simulink model "launch_control"  (R2023b)
settings: Solver=VariableStepAuto  StartTime=0.0  StopTime=10.0  RelTol=1e-3
settings Model: Creator=no  LastModifiedBy=no

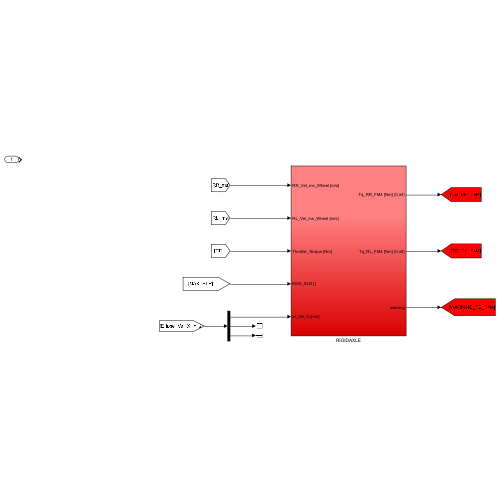
[thumbnail: Simulink's stored preview of the top-level diagram]
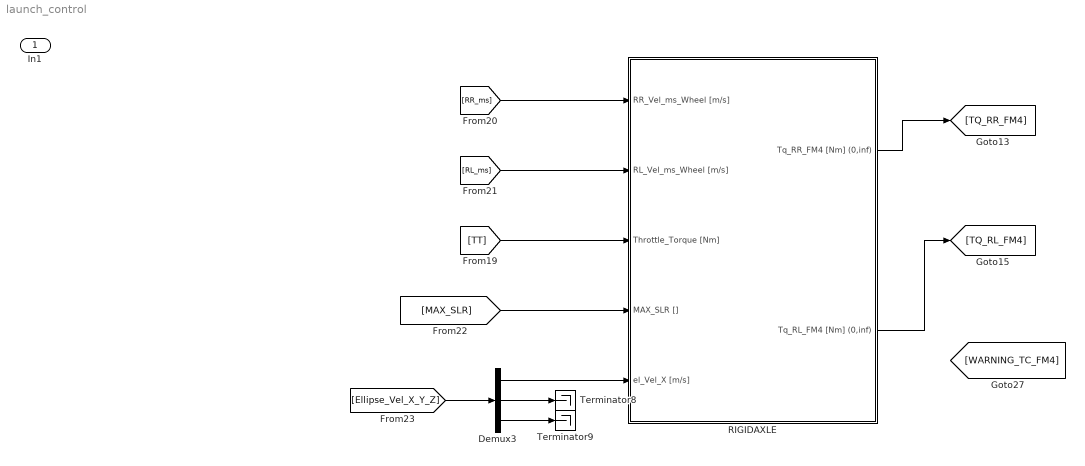
== system launch_control ==
  In1 : Inport
  Demux3 : Demux  Outputs=3
  RIGIDAXLE : Subsystem
  Terminator8 : Terminator
  Terminator9 : Terminator
  wires:
  [TT] -> RIGIDAXLE/3(Throttle_Torque [Nm])
  ? -> [WARNING_TC_FM4]
  [RL_ms] -> RIGIDAXLE/2(RL_Vel_ms_Wheel [m/s])
  RIGIDAXLE/1(Tq_RR_FM4 [Nm] (0,inf)) -> [TQ_RR_FM4]
  [RR_ms] -> RIGIDAXLE/1(RR_Vel_ms_Wheel [m/s])
  Demux3/1 -> RIGIDAXLE/5(el_Vel_X [m/s])
  Demux3/3 -> Terminator9/1
  Demux3/2 -> Terminator8/1
  [Ellipse_Vel_X_Y_Z] -> Demux3/1
  [MAX_SLR] -> RIGIDAXLE/4(MAX_SLR [])
  RIGIDAXLE/2(Tq_RL_FM4 [Nm] (0,inf)) -> [TQ_RL_FM4]

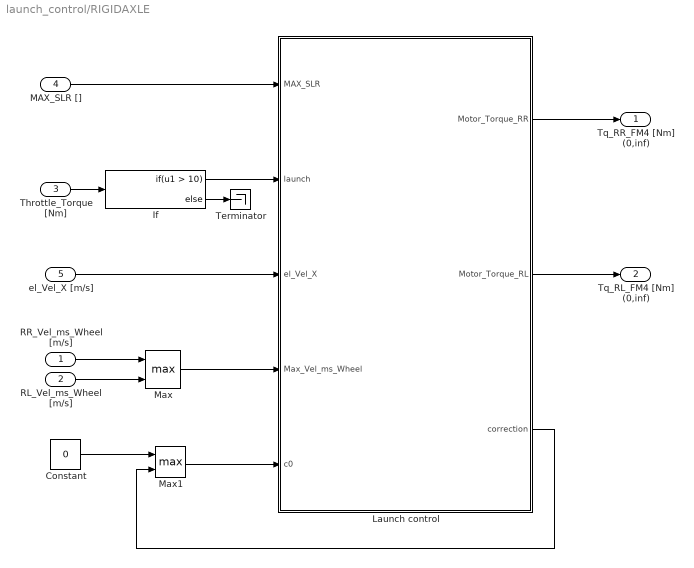
== system launch_control/RIGIDAXLE ==
  RR_Vel_ms_Wheel [m/s] : Inport
  RL_Vel_ms_Wheel [m/s] : Inport  Port=2
  Throttle_Torque [Nm] : Inport  Port=3
  MAX_SLR [] : Inport  Port=4
  el_Vel_X [m/s] : Inport  Port=5
  Constant : Constant  Value=0
  If : If  IfExpression=u1 > 10
  Launch control : MATLAB Function  TreatAsAtomicUnit=on
  Max : MinMax  Function=max  Inputs=2
  Max1 : MinMax  Function=max  Inputs=2
  Terminator : Terminator
  Tq_RR_FM4 [Nm] (0,inf) : Outport  VectorParamsAs1DForOutWhenUnconnected=off
  Tq_RL_FM4 [Nm] (0,inf) : Outport  Port=2  VectorParamsAs1DForOutWhenUnconnected=off
  wires:
  RR_Vel_ms_Wheel [m/s]/1 -> Max/1
  Launch control/1(Motor_Torque_RR) -> Tq_RR_FM4 [Nm] (0,inf)/1
  Launch control/3(correction) -> Max1/2
  Constant/1 -> Max1/1
  Max1/1 -> Launch control/5(c0)
  Launch control/2(Motor_Torque_RL) -> Tq_RL_FM4 [Nm] (0,inf)/1
  Max/1 -> Launch control/4(Max_Vel_ms_Wheel)
  RL_Vel_ms_Wheel [m/s]/1 -> Max/2
  MAX_SLR []/1 -> Launch control/1(MAX_SLR)
  el_Vel_X [m/s]/1 -> Launch control/3(el_Vel_X)
  Throttle_Torque [Nm]/1 -> If/1
  If/1 -> Launch control/2(launch)
  If/2 -> Terminator/1

== matlab function launch_control/RIGIDAXLE/Launch control ==
  data: MAX_SLR input; launch input; Motor_Torque_RR output; Motor_Torque_RL output; el_Vel_X input; Max_Vel_ms_Wheel input; correction output; c0 input
function [Motor_Torque_RR, Motor_Torque_RL, correction] = LAUNCH_CONTROL(MAX_SLR, launch, el_Vel_X, Max_Vel_ms_Wheel, c0)
if launch
    Motor_Torque = 27;
    % SLIP RATIO CALCULATIONS
    % calculate slip ratio
    SLR = (Max_Vel_ms_Wheel/el_Vel_X);

    % CHECK FOR EXCESIVE SLIPPING
    % SLIP RATIO LESSER THAN MAXIMUM SLIP RATIO => apply max torque times throttle factor
    if(SLR<MAX_SLR)
        Motor_Torque_RR = Motor_Torque;
        Motor_Torque_RL = Motor_Torque;
        correction = 0; %set correction to 0 as tyre is not slipping
        return;
    else
        % TYRE SLIPPING => TC INTERVENES
        % LOOK FOR THE PREVIOUS CORRECTION [Nm]
        if(c0 == 0) % NOT SLIPPING PREVIOUSLY
            correction = 1; % [INTERVAL TO BE DETERMINED] set the correction to the torque we want to substract
            Motor_Torque_RR = Motor_Torque-correction; % substract the correction from the torque to apply
            Motor_Torque_RL = Motor_Torque-correction;
            return;
        else % TYRE SLIPPING PREVIOUSLY
            correction = c0 + 1; % [INTERVAL TO BE DETERMINED] set the correction to the torque we want to substract + previous corrections
            Motor_Torque_RR = Motor_Torque-correction; % substract the correction from the torque to apply
            Motor_Torque_RL = Motor_Torque-correction;
            return;
        end
    end
end
end
